simulink model "Danna"  (R2022a)
settings: Solver=VariableStepAuto  StartTime=0.0  StopTime=inf  RelTol=1e-3
undefined symbols (not defined in the file or in its folder): Angular, Linear
libraries: robotlib x5
settings Model: Creator=admin  LastModifiedBy=admin

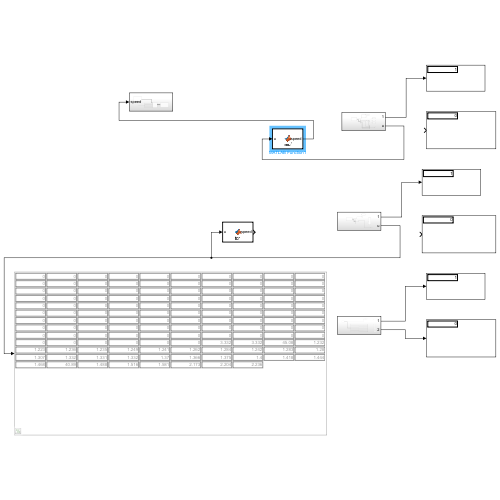
[thumbnail: Simulink's stored preview of the top-level diagram]
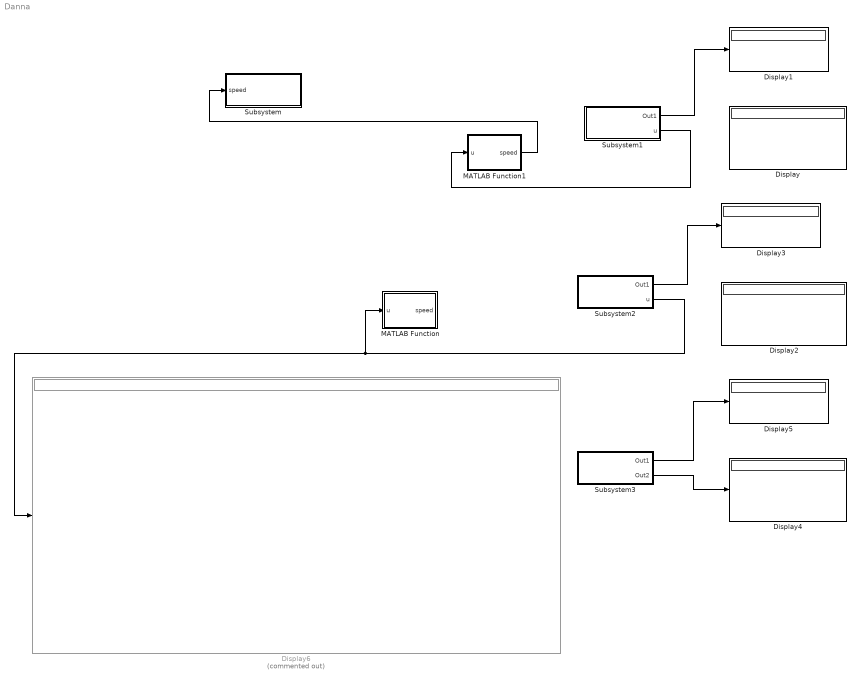
== system Danna ==
  Display{,1..5} (6 alike) : Display
  Display6 : Display  Commented=on
  MATLAB Function : MATLAB Function  TreatAsAtomicUnit=on
  MATLAB Function1 : MATLAB Function  TreatAsAtomicUnit=on
  Subsystem : Subsystem
  Subsystem1 : Subsystem
  Subsystem2 : Subsystem
  Subsystem3 : Subsystem
  wires:
  Subsystem1/1(Out1) -> Display1/1
  Subsystem1/2(u) -> MATLAB Function1/1(u)
  Subsystem2/2(u) -> Display6/1, MATLAB Function/1(u)
  Subsystem2/1(Out1) -> Display3/1
  Subsystem3/2(Out2) -> Display4/1
  Subsystem3/1(Out1) -> Display5/1
  MATLAB Function1/1(speed) -> Subsystem/1(speed)

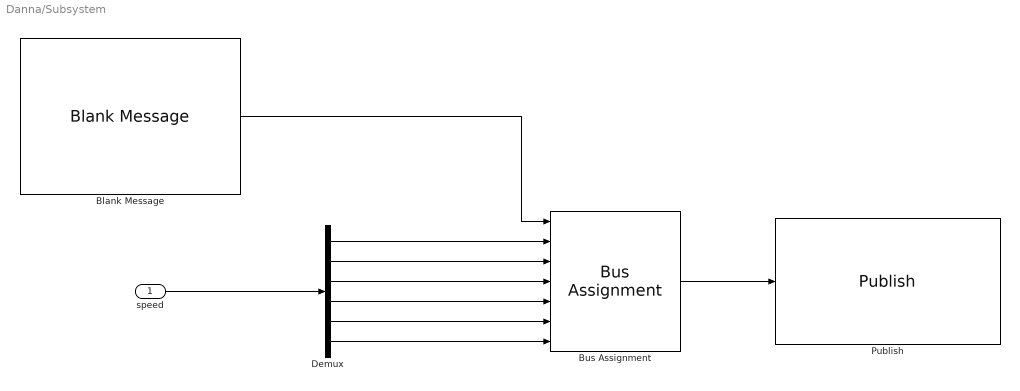
== system Danna/Subsystem ==
  speed : Inport
  Blank Message : robotlib/Blank Message  messageClass=Message  entityType=geometry_msgs/Twist  messageType=geometry_msgs/Twist  SampleTime=inf  legacyBusStruct=off
  Bus Assignment : BusAssignment  AssignedSignals=Linear.X,Angular.Z,Angular.Y,Angular.X,Linear.Y,Linear.Z
  Demux : Demux  Outputs=6
  Publish : robotlib/Publish  topicSource=Specify your own  topic=/cmd_vel  messageType=geometry_msgs/Twist  legacyBusStruct=off  messageQueueLength=1
  wires:
  Blank Message/1 -> Bus Assignment/1
  Demux/1 -> Bus Assignment/2
  Demux/2 -> Bus Assignment/3
  Demux/3 -> Bus Assignment/4
  Demux/4 -> Bus Assignment/5
  Demux/5 -> Bus Assignment/6
  Demux/6 -> Bus Assignment/7
  speed/1 -> Demux/1
  Bus Assignment/1 -> Publish/1

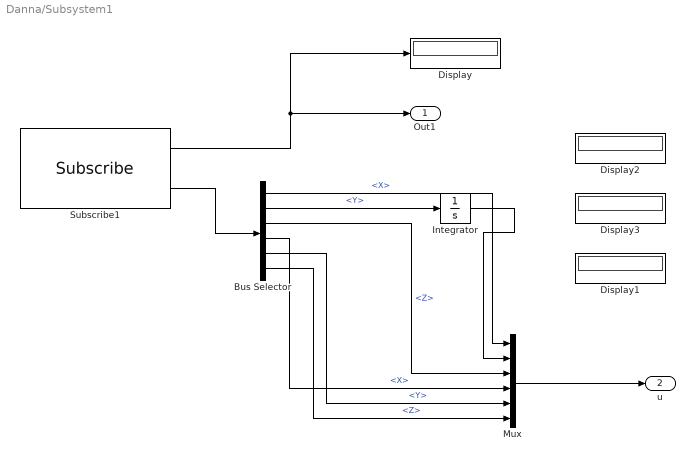
== system Danna/Subsystem1 ==
  Bus Selector : BusSelector  OutputSignals=AngularVelocity.X,AngularVelocity.Y,AngularVelocity.Z,LinearAcceleration.X,LinearAcceleration.Y,LinearAcceleration.Z
  Display{,1..3} (4 alike) : Display
  Integrator : Integrator
  Mux : Mux  Inputs=6
  Subscribe1 : robotlib/Subscribe  topicSource=Specify your own  topic=/imu  messageType=sensor_msgs/Imu  SampleTime=0.1  legacyBusStruct=off  messageQueueLength=1
  Out1 : Outport
  u : Outport  Port=2
  wires:
  Bus Selector/1 -> Mux/1  "<X>"
  Bus Selector/6 -> Mux/6  "<Z>"
  Mux/1 -> u/1
  Bus Selector/3 -> Mux/3  "<Z>"
  Bus Selector/5 -> Mux/5  "<Y>"
  Bus Selector/4 -> Mux/4  "<X>"
  Subscribe1/1 -> Display/1, Out1/1
  Subscribe1/2 -> Bus Selector/1
  Bus Selector/2 -> Integrator/1  "<Y>"
  Integrator/1 -> Mux/2

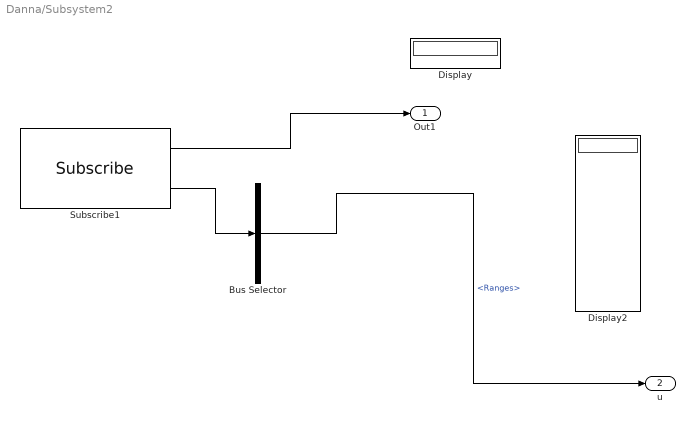
== system Danna/Subsystem2 ==
  Bus Selector : BusSelector  OutputSignals=Ranges
  Display : Display
  Display2 : Display
  Subscribe1 : robotlib/Subscribe  topicSource=Specify your own  topic=/scan  messageType=sensor_msgs/LaserScan  SampleTime=0.01  legacyBusStruct=off  messageQueueLength=1
  Out1 : Outport
  u : Outport  Port=2
  wires:
  Bus Selector/1 -> u/1  "<Ranges>"
  Subscribe1/1 -> Out1/1
  Subscribe1/2 -> Bus Selector/1

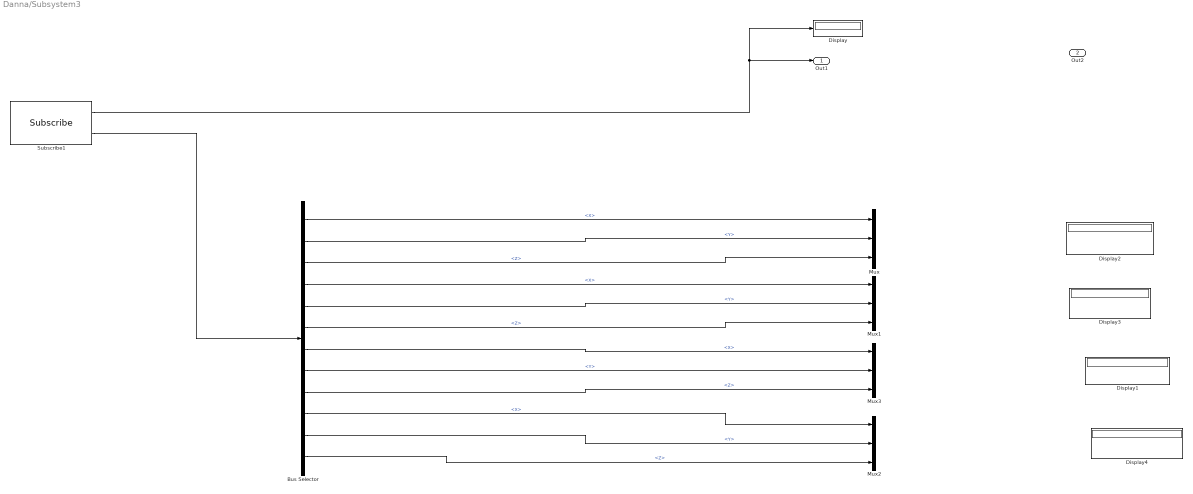
== system Danna/Subsystem3 ==
  Bus Selector : BusSelector  OutputSignals=Pose.Pose.Position.X,Pose.Pose.Position.Y,Pose.Pose.Position.Z,Pose.Pose.Orientation.X,Pose.Pose.Orientation.Y,Pose.Pose.Orientation.Z,Twist.Twist.Linear.X,Twist.Twist.Linear.Y,Twist.Twist.Linear.Z,Twist.Twist.Angular.X,Twist.Twist.Angular.Y,Twist.Twist.Angular.Z
  Display{,1..4} (5 alike) : Display
  Mux{,1..3} (4 alike) : Mux  Inputs=3
  Subscribe1 : robotlib/Subscribe  topicSource=Specify your own  topic=/odom  messageType=nav_msgs/Odometry  SampleTime=0.1  legacyBusStruct=off  messageQueueLength=1
  Out1 : Outport
  Out2 : Outport  Port=2
  wires:
  Subscribe1/1 -> Display/1, Out1/1
  Subscribe1/2 -> Bus Selector/1
  Bus Selector/1 -> Mux/1  "<X>"
  Bus Selector/2 -> Mux/2  "<Y>"
  Bus Selector/3 -> Mux/3  "<Z>"
  Bus Selector/4 -> Mux1/1  "<X>"
  Bus Selector/5 -> Mux1/2  "<Y>"
  Bus Selector/6 -> Mux1/3  "<Z>"
  Bus Selector/7 -> Mux3/1  "<X>"
  Bus Selector/8 -> Mux3/2  "<Y>"
  Bus Selector/9 -> Mux3/3  "<Z>"
  Bus Selector/10 -> Mux2/1  "<X>"
  Bus Selector/11 -> Mux2/2  "<Y>"
  Bus Selector/12 -> Mux2/3  "<Z>"

== matlab function Danna/MATLAB Function ==
  data: u input; speed output
function speed = fcn(u)

    figure(1)
    plot(u)
    
    x=u(90:100);
    M=mean(x,'all');
    
    if(M<10);
        speed = [0,0,0,0,0,0]
    else;
        speed=[0,0,0,0,0,0]
    end

end

== matlab function Danna/MATLAB Function1 ==
  data: u input; speed output
function speed  = imuf(u)

%{
    if(u(2)==0);
        speed=[0.05,0,0,0,0,0];
    elseif(u(2)>0);
        speed=[0.02,0,0,0,0,0];
    else;
        speed=[0.1,0,0,0,0,0];
    end
%}
    if(u(2)>0.1);
        speed=[0.02,0,0,0,0,0];
    elseif(u(2)<-0.1);
        speed=[0.1,0,0,0,0,0];
    else;
        speed=[0.05,0,0,0,0,0];
    end

end
